simulink model "wing"  (Simulink 6.6)
settings: Solver=ode23s  StartTime=0.0  StopTime=2  RelTol=1e-3
undefined symbols (not defined in the file or in its folder): wing_control
libraries: simulink x1
settings Model: Creator=nsz  LastModifiedBy=nsz  ExtModeTrigMode=oneshot  ExtModeArmWhenConnect=off  ExtModeAutoUpdateStatusClock=off
settings DataIOCC: LimitDataPoints=off  SaveOutput=off  SaveTime=off
settings OptimizationCC: BooleanDataType=off  InlineInvariantSignals=on
settings DebuggingCC: SignalResolutionControl=TryResolveAllWithWarning  SolverPrmCheckMsg=none  MultiTaskDSMMsg=warning  MultiTaskCondExecSysMsg=none  StrictBusMsg=None
settings HardwareCC: TargetUnknown=on
settings RTWCC: IncludeERTFirstTime=on
settings GRTTargetCC: ModelReferenceCompliant=off  MatFileLogging=off

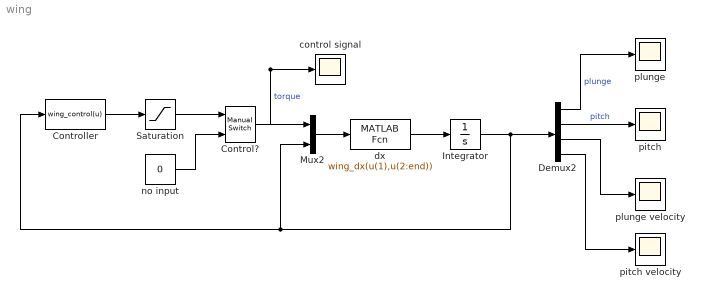
== system wing ==
  Control? : simulink/Signal Routing/Manual Switch  SystemSampleTime=-1  sw=1  action=0  varsize=off
  Controller : MATLABFcn  MATLABFcn=wing_control(u)  OutputDimensions=1
  Demux2 : Demux
  Integrator : Integrator  InitialCondition=[0.01,0.1,0,0]
  Mux2 : Mux  Inputs=2
  Saturation : Saturate  UpperLimit=100  LowerLimit=-100
  control signal : Scope
      settings: YMin=-100  YMax=100  SaveName=ScopeData3
  dx : MATLABFcn  MATLABFcn=wing_dx(u(1),u(2:end))  OutputDimensions=4
  no input : Constant  Value=0
  pitch : Scope
      settings: YMin=-0.01  YMax=0.1  SaveName=ScopeData5
  pitch velocity : Scope
      settings: YMin=-0.045  YMax=0.055  SaveName=ScopeData2
  plunge : Scope
      settings: YMin=-0.05  YMax=0.025  SaveName=ScopeData4
  plunge velocity : Scope
      settings: YMin=-0.45  YMax=0.55
  wires:
  Mux2/1 -> dx/1
  dx/1 -> Integrator/1
  Demux2/1 -> plunge/1  "plunge"
  Demux2/2 -> pitch/1  "pitch"
  Integrator/1 -> Demux2/1, Mux2/2, Controller/1
  Demux2/3 -> plunge velocity/1
  no input/1 -> Control?/2
  Demux2/4 -> pitch velocity/1
  Control?/1 -> Mux2/1, control signal/1  "torque"
  Controller/1 -> Saturation/1
  Saturation/1 -> Control?/1
